simulink model "Sim2"  (R2016b)
settings: Solver=VariableStepAuto  StartTime=0.0  StopTime=1000  FixedStep=0.01  RelTol=1e-3
undefined symbols (not defined in the file or in its folder): DiscIntNeverNeededParam, i
libraries: commsink2 x1, dspsrcs4 x1, commrandsrc3 x1
settings Model: Creator=ASUS  LastModifiedBy=ASUS

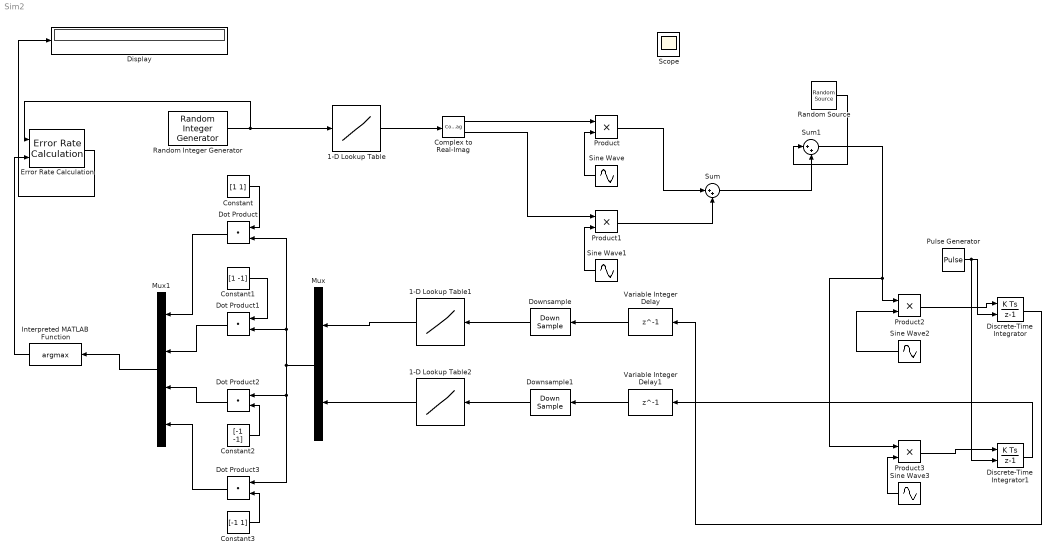
== system Sim2 ==
  1-D Lookup Table : Lookup_n-D  NumberOfTableDimensions=1  BreakpointsForDimension1=[0 1 2 3]  Table=[1+i 1-i -1-i -1+i]  InternalRulePriority=Speed  RndMeth=Simplest  InputSameDT=on
  1-D Lookup Table1 : Lookup_n-D  NumberOfTableDimensions=1  BreakpointsForDimension1=[-10 -eps eps 10]  Table=[-1 -1 1 1]  InternalRulePriority=Speed  RndMeth=Simplest  InputSameDT=on
  1-D Lookup Table2 : Lookup_n-D  NumberOfTableDimensions=1  BreakpointsForDimension1=[-10 -eps eps 10]  Table=[-1 -1 1 1]  InternalRulePriority=Speed  RndMeth=Simplest  InputSameDT=on
  Complex to Real-Imag : ComplexToRealImag
  Constant : Constant  Value=[1 1]
  Constant1 : Constant  Value=[1 -1]
  Constant2 : Constant  Value=[-1 -1]
  Constant3 : Constant  Value=[-1 1]
  Discrete-Time Integrator : DiscreteIntegrator  ExternalReset=rising  InitialConditionSetting=State (most efficient)  SampleTime=-1  ICPrevOutput=DiscIntNeverNeededParam  ICPrevScaledInput=DiscIntNeverNeededParam
  Discrete-Time Integrator1 : DiscreteIntegrator  ExternalReset=rising  InitialConditionSetting=State (most efficient)  SampleTime=-1  ICPrevOutput=DiscIntNeverNeededParam  ICPrevScaledInput=DiscIntNeverNeededParam
  Display : Display
  Dot Product{,1..3} (4 alike) : DotProduct  InputSameDT=on  OutDataTypeStr=Inherit: Inherit via internal rule
  Downsample : DownSample  N=100  RateOptions=Allow multirate processing
  Downsample1 : DownSample  N=100  RateOptions=Allow multirate processing
  Error Rate Calculation : commsink2/Error Rate Calculation  N=1  st_delay=0  cp_mode=Entire frame  subframe=[]  PMode=Port  WsName=ErrorVec  RsMode2=off  stop=off  numErr=100  maxBits=1e6
  Interpreted MATLAB Function : MATLABFcn  MATLABFcn=argmax
  Mux : Mux  Inputs=2
  Mux1 : Mux
  Product{,1..3} (4 alike) : Product
  Pulse Generator : DiscretePulseGenerator  Period=100  PulseWidth=50  SampleTime=.01
  Random Source : dspsrcs4/Random Source  SrcType=Uniform  NormMethod=Ziggurat  CltLength=12  MinVal=0  MaxVal=1  MeanVal=0  VarVal=1  RepMode=Not repeatable  rawSeed=1  IsInherit=off  SampMode=Discrete  SampTime=1  SampFrame=1  DataType=Double  OutComplex=Real  OutputFrames=off
  Random Integer Generator : commrandsrc3/Random Integer Generator  SetSize=4  SeedSource=Auto  Seed=0  SampleTime=1  SamplesPerFrame=1  OutputDataType=double  SimulateUsing=Interpreted execution
  Scope : Scope
  Sine Wave : Sin  Amplitude=sqrt(20)  Frequency=10  SampleTime=0.01
  Sine Wave1 : Sin  Amplitude=sqrt(20)  Frequency=10  Phase=pi/2  SampleTime=0.01
  Sine Wave2 : Sin  Amplitude=sqrt(20)  Frequency=10  SampleTime=0.01
  Sine Wave3 : Sin  Amplitude=sqrt(20)  Frequency=10  Phase=pi/2  SampleTime=0.01
  Sum : Sum  Inputs=|++
  Sum1 : Sum  Inputs=|++
  Variable Integer Delay : Delay  DelayLength=1
  Variable Integer Delay1 : Delay  DelayLength=1
  wires:
  Random Integer Generator/1 -> Error Rate Calculation/1, 1-D Lookup Table/1
  1-D Lookup Table/1 -> Complex to Real-Imag/1
  Sine Wave/1 -> Product/2
  Sine Wave1/1 -> Product1/2
  Complex to Real-Imag/2 -> Product1/1
  Product1/1 -> Sum/2
  Product/1 -> Sum/1
  Sum/1 -> Sum1/2
  Sine Wave2/1 -> Product2/2
  Sine Wave3/1 -> Product3/2
  Sum1/1 -> Product3/1, Product2/1
  Product3/1 -> Discrete-Time Integrator1/1
  Product2/1 -> Discrete-Time Integrator/1
  Discrete-Time Integrator/1 -> Variable Integer Delay/1
  Discrete-Time Integrator1/1 -> Variable Integer Delay1/1
  Variable Integer Delay/1 -> Downsample/1
  Variable Integer Delay1/1 -> Downsample1/1
  Pulse Generator/1 -> Discrete-Time Integrator/2, Discrete-Time Integrator1/2
  Downsample/1 -> 1-D Lookup Table1/1
  Downsample1/1 -> 1-D Lookup Table2/1
  1-D Lookup Table1/1 -> Mux/1
  1-D Lookup Table2/1 -> Mux/2
  Mux/1 -> Dot Product3/1, Dot Product2/1, Dot Product/2, Dot Product1/2
  Constant3/1 -> Dot Product3/2
  Constant2/1 -> Dot Product2/2
  Constant1/1 -> Dot Product1/1
  Constant/1 -> Dot Product/1
  Dot Product/1 -> Mux1/1
  Dot Product1/1 -> Mux1/2
  Dot Product2/1 -> Mux1/3
  Dot Product3/1 -> Mux1/4
  Mux1/1 -> Interpreted MATLAB Function/1
  Interpreted MATLAB Function/1 -> Error Rate Calculation/2
  Error Rate Calculation/1 -> Display/1
  Random Source/1 -> Sum1/1
  Complex to Real-Imag/1 -> Product/1
